simulink model "B5_simulation_paparazzi"  (R2021b)
settings: Solver=VariableStepAuto  StartTime=0.0  StopTime=5.5  FixedStep=0.002  RelTol=1e-3
values from neighbouring files (symbols this model uses):
  coef_sim_1 = tf_des_d.Denominator{1}(2)    [A11_setup_script_pprz.m]    (also in A1_setup_script.m; A6_slow_actuator.m)
  coef_sim_2 = tf_des_d.Numerator{1}(2)    [A11_setup_script_pprz.m]    (also in A1_setup_script.m; A6_slow_actuator.m)
  coeff = 1    [A11_setup_script_pprz.m]    (also in A12_sim_multi_run.m = coeff_list(i))
  doublet_mag = - 0.15    (= -0.15)    [A11_setup_script_pprz.m]    (also in A1_setup_script.m)
  doublet_time = 6    [A11_setup_script_pprz.m]    (also in A1_setup_script.m)
  f_8 = 1    [A11_setup_script_pprz.m]    (also in A1_setup_script.m)
  FILT_CUTOFF = 2*pi*5    (= 31.4159265359)    [A11_setup_script_pprz.m]    (also in A1_setup_script.m)
  FILTER = 1    [A11_setup_script_pprz.m]    (also in A1_setup_script.m)
  G1 = inv(I)*G1_r    [A10_simple_plant.m]    (also in A11_setup_script_pprz.m = G1/scale; A1_setup_script.m = [G1;G1_T])
  G2 = G2/scale    [A11_setup_script_pprz.m]    (also in A1_setup_script.m = (1/sampling_time)*inv(I)*(G2_r))
  h_plate = 0.3    [A11_setup_script_pprz.m]    (also in A1_setup_script.m = 0.16)
  I = eye(3,3)    [A10_simple_plant.m]    (also in A11_setup_script_pprz.m; A1_setup_script.m; A2_B_matrix_generation_symbolic.m = [Ixx 0 0; A3_B_matrix_generation_symbolic_cascaded.m = [Ixx 0 0)
  Iyy = 0.0008    [A11_setup_script_pprz.m]    (also in A1_setup_script.m = 0.0015)
  K = 7    [A11_setup_script_pprz.m]    (also in A1_setup_script.m = 10)
  K_act = 50    [A10_simple_plant.m]    (also in A11_setup_script_pprz.m = 20; A1_setup_script.m = 20)
  K_d = 15    [A11_setup_script_pprz.m]    (also in A1_setup_script.m = 25)
  K_dd = K_act    (= 20)    [A11_setup_script_pprz.m]    (also in A1_setup_script.m)
  K_ec = 50    [A11_setup_script_pprz.m]    (also in A1_setup_script.m = 251)
  K_ec_d = 13    [A11_setup_script_pprz.m]    (also in A1_setup_script.m = 25)
  K_ec_d_u = 1.5    [A11_setup_script_pprz.m]    (also in A1_setup_script.m = 5)
  K_ec_d_v = 1.5    [A11_setup_script_pprz.m]    (also in A1_setup_script.m = 5)
  K_ec_dd = 9    [A11_setup_script_pprz.m]    (also in A1_setup_script.m = 45)
  K_ec_i = 0    [A11_setup_script_pprz.m]    (also in A1_setup_script.m = 380)
  K_ec_u = 1.5    [A11_setup_script_pprz.m]    (also in A1_setup_script.m = 5)
  K_ec_v = 1.5    [A11_setup_script_pprz.m]    (also in A1_setup_script.m = 5)
  K_t = 0.0005    [A10_simple_plant.m]    (also in A11_setup_script_pprz.m = 6.557e-08; A1_setup_script.m = 6.557e-08)
  K_u = 1.0    (= 1)    [A11_setup_script_pprz.m]    (also in A1_setup_script.m = 1.5)
  K_u_d = 2.5    [A11_setup_script_pprz.m]    (also in A1_setup_script.m = 7)
  K_v = 1.0    (= 1)    [A11_setup_script_pprz.m]    (also in A1_setup_script.m = 1.5)
  K_v_d = 2.5    [A11_setup_script_pprz.m]    (also in A1_setup_script.m = 7)
  K_w = 1.0    (= 1)    [A11_setup_script_pprz.m]    (also in A1_setup_script.m = 4.5)
  K_w_d = 2.5    [A11_setup_script_pprz.m]    (also in A1_setup_script.m = 7)
  l_plate = 0.1    [A11_setup_script_pprz.m]    (also in A1_setup_script.m = 0.11)
  m = 0.4    [A10_simple_plant.m]    (also in A11_setup_script_pprz.m; A1_setup_script.m)
  NOISE = 0    [A11_setup_script_pprz.m]    (also in A1_setup_script.m)
  NOISE_ACC = 0.00005    (= 5e-05)    [A11_setup_script_pprz.m]    (also in A1_setup_script.m)
  NOISE_GYRO = 0.00005    (= 5e-05)    [A11_setup_script_pprz.m]    (also in A1_setup_script.m)
  NOISE_RPM = 200    [A11_setup_script_pprz.m]    (also in A1_setup_script.m)
  omega_des = 20.00    (= 20)    [A11_setup_script_pprz.m]    (also in A1_setup_script.m; A6_slow_actuator.m = 49)
  sampling_time = 1/frequency    (= 0.002)    [A11_setup_script_pprz.m]    (also in A12_sim_multi_run.m; A1_setup_script.m; A6_slow_actuator.m)
  scale_8 = 1.6    [A11_setup_script_pprz.m]    (also in A1_setup_script.m)
  start_8 = 2    [A11_setup_script_pprz.m]    (also in A1_setup_script.m)
  start_time = 2    [A11_setup_script_pprz.m]    (also in A1_setup_script.m = 1)
  t_8 = 10    [A11_setup_script_pprz.m]    (also in A1_setup_script.m)
  w_plate = 0.3    [A11_setup_script_pprz.m]    (also in A1_setup_script.m = 0.36)
undefined symbols (not defined in the file or in its folder): DiscIntNeverNeededParam
libraries: simulink x11, cstblocks x9, dspinverses x8, dspmathops x4, dspstat3 x4, aerolibutil x3, sharedutil x2, aerolibanim x1
(part 4 of 5)

== system B5_simulation_paparazzi/Model Block Complementary Filters/Plant and State Estimation/Complementary Filter1/Butterworth Lowpass 2nd Order1 ==
  In : Inport
  Constant : Constant  Value=FILTER  SampleTime=sampling_time
  Merge : Merge
  Switch Case : SwitchCase
  Switch Case Action Subsystem : Subsystem  TreatAsAtomicUnit=on
  Switch Case Action Subsystem1 : Subsystem  TreatAsAtomicUnit=on
  Out : Outport
  wires:
  Merge/1 -> Out/1
  Switch Case Action Subsystem/1(Out1) -> Merge/1
  Constant/1 -> Switch Case/1
  Switch Case Action Subsystem1/1(Out1) -> Merge/2
  Switch Case/2 -> Switch Case Action Subsystem1/Action
  In/1 -> Switch Case Action Subsystem/1(In1), Switch Case Action Subsystem1/1(In1)
  Switch Case/1 -> Switch Case Action Subsystem/Action

== system B5_simulation_paparazzi/Model Block Complementary Filters/Plant and State Estimation/Complementary Filter1/Butterworth Lowpass 2nd Order2 ==
  In : Inport
  Constant : Constant  Value=FILTER  SampleTime=sampling_time
  Merge : Merge
  Switch Case : SwitchCase
  Switch Case Action Subsystem : Subsystem  TreatAsAtomicUnit=on
  Switch Case Action Subsystem1 : Subsystem  TreatAsAtomicUnit=on
  Out : Outport
  wires:
  Merge/1 -> Out/1
  Switch Case Action Subsystem/1(Out1) -> Merge/1
  Constant/1 -> Switch Case/1
  Switch Case Action Subsystem1/1(Out1) -> Merge/2
  Switch Case/2 -> Switch Case Action Subsystem1/Action
  In/1 -> Switch Case Action Subsystem/1(In1), Switch Case Action Subsystem1/1(In1)
  Switch Case/1 -> Switch Case Action Subsystem/Action

== system B5_simulation_paparazzi/Model Block Complementary Filters/Plant and State Estimation/Noise Acc/Switch Case Action Subsystem ==
  Action Port : ActionPort  ActionPortLabel=case [ 1 ]:
  Acc Noise : simulink/Sources/Band-Limited White Noise  Cov=[NOISE_ACC]  Ts=sampling_time  seed=[23341]
  Out1 : Outport
  wires:
  Acc Noise/1 -> Out1/1

== system B5_simulation_paparazzi/Model Block Complementary Filters/Plant and State Estimation/Noise Acc/Switch Case Action Subsystem1 ==
  Action Port : ActionPort  ActionPortLabel=default:
  Constant : Constant  Value=0  SampleTime=sampling_time
  Out1 : Outport
  wires:
  Constant/1 -> Out1/1

== system B5_simulation_paparazzi/Model Block Complementary Filters/Plant and State Estimation/Noise Gyro/Switch Case Action Subsystem ==
  Action Port : ActionPort  ActionPortLabel=case [ 1 ]:
  Gyro Noise : simulink/Sources/Band-Limited White Noise  Cov=[NOISE_GYRO]  Ts=sampling_time  seed=[23341]
  Out1 : Outport
  wires:
  Gyro Noise/1 -> Out1/1

== system B5_simulation_paparazzi/Model Block Complementary Filters/Plant and State Estimation/Noise Gyro/Switch Case Action Subsystem1 ==
  Action Port : ActionPort  ActionPortLabel=default:
  Constant : Constant  Value=0  SampleTime=sampling_time
  Out1 : Outport
  wires:
  Constant/1 -> Out1/1

== system B5_simulation_paparazzi/Model Block Complementary Filters/Plant and State Estimation/Plant Dynamics Continuous/Disturbance Block ==
  Step : Step  Time=2  After=60  SampleTime=0
  Sum : Sum  Inputs=|++
  Total Disturbance : Outport
  wires:
  Step/1 -> Sum/1
  Sum/1 -> Total Disturbance/1

== system B5_simulation_paparazzi/Model Block Complementary Filters/Plant and State Estimation/Plant Dynamics Continuous/Omega_I_Omega1 ==
  pqr_body : Inport
  Inertia : Inport  Port=2
  3x3 Cross Product : sharedutil/3x3 Cross Product  aMode=aMode
      settings: SourceProductBaseCode=AE,PW,DR,MT,UV,VE
  Matrix Multiply1 : Product  Multiplication=Matrix(*)
  Final product : Outport
  wires:
  Inertia/1 -> Matrix Multiply1/1
  Matrix Multiply1/1 -> 3x3 Cross Product/2
  3x3 Cross Product/1 -> Final product/1
  pqr_body/1 -> 3x3 Cross Product/1, Matrix Multiply1/2

== system B5_simulation_paparazzi/Model Block Complementary Filters/Simple INDI/INTERNAL REFERENCE MODEL ATTITUDE/body rates to euler rates ==
  p : Inport
  q : Inport  Port=2
  r : Inport  Port=3
  Demux : Demux  Outputs=3
  Matrix Multiply : Product  Multiplication=Matrix(*)
  Mux : Mux  Inputs=3
  phi_dot : Outport
  theta_dot : Outport  Port=2
  psi_dot : Outport  Port=3
  wires:
  p/1 -> Mux/1
  q/1 -> Mux/2
  r/1 -> Mux/3
  [T_discr] -> Matrix Multiply/1
  Mux/1 -> Matrix Multiply/2
  Matrix Multiply/1 -> Demux/1
  Demux/3 -> psi_dot/1
  Demux/2 -> theta_dot/1
  Demux/1 -> phi_dot/1

== system B5_simulation_paparazzi/Model Block Complementary Filters/Simple INDI/INTERNAL REFERENCE MODEL ATTITUDE/euler rates to body rates ==
  phi_dot : Inport
  theta_dot : Inport  Port=2
  psi_dot : Inport  Port=3
  Demux : Demux  Outputs=3
  Matrix Multiply : Product  Multiplication=Matrix(*)
  Mux : Mux  Inputs=3
  p : Outport
  q : Outport  Port=2
  r : Outport  Port=3
  wires:
  phi_dot/1 -> Mux/1
  theta_dot/1 -> Mux/2
  psi_dot/1 -> Mux/3
  [R_discr] -> Matrix Multiply/1
  Mux/1 -> Matrix Multiply/2
  Matrix Multiply/1 -> Demux/1
  Demux/3 -> r/1
  Demux/2 -> q/1
  Demux/1 -> p/1

== system B5_simulation_paparazzi/Model Block Normal Filters/Continuous Actuator Dynamics/Butterworth Lowpass 2nd Order1/Switch Case Action Subsystem ==
  In1 : Inport
  Action Port : ActionPort  ActionPortLabel=case [ 1 ]:
  Constant5 : Constant  Value=FILT_CUTOFF  SampleTime=sampling_time
  Lowpass2 : cstblocks/Linear Parameter Varying/Discrete Varying Lowpass  N=2  w0=0  Ts=sampling_time
      settings: SourceProductBaseCode=CT
  Out1 : Outport
  wires:
  Constant5/1 -> Lowpass2/2
  In1/1 -> Lowpass2/1
  Lowpass2/1 -> Out1/1

== system B5_simulation_paparazzi/Model Block Normal Filters/Continuous Actuator Dynamics/Butterworth Lowpass 2nd Order1/Switch Case Action Subsystem1 ==
  In1 : Inport
  Action Port : ActionPort  ActionPortLabel=default:
  Out1 : Outport
  wires:
  In1/1 -> Out1/1

== system B5_simulation_paparazzi/Model Block Normal Filters/Continuous Actuator Dynamics/Noise RPM/Switch Case Action Subsystem ==
  Action Port : ActionPort  ActionPortLabel=case [ 1 ]:
  RPM Noise : simulink/Sources/Band-Limited White Noise  Cov=[NOISE_RPM]  Ts=sampling_time  seed=[23341]
  Out1 : Outport
  wires:
  RPM Noise/1 -> Out1/1

== system B5_simulation_paparazzi/Model Block Normal Filters/Continuous Actuator Dynamics/Noise RPM/Switch Case Action Subsystem1 ==
  Action Port : ActionPort  ActionPortLabel=default:
  Constant : Constant  Value=0  SampleTime=sampling_time
  Out1 : Outport
  wires:
  Constant/1 -> Out1/1

== system B5_simulation_paparazzi/Model Block Normal Filters/Extended INDI/INTERNAL REFERENCE MODEL ATTITUDE/body rates to euler rates ==
  p : Inport
  q : Inport  Port=2
  r : Inport  Port=3
  Demux : Demux  Outputs=3
  Matrix Multiply : Product  Multiplication=Matrix(*)
  Mux : Mux  Inputs=3
  phi_dot : Outport
  theta_dot : Outport  Port=2
  psi_dot : Outport  Port=3
  wires:
  p/1 -> Mux/1
  q/1 -> Mux/2
  r/1 -> Mux/3
  [T_discr] -> Matrix Multiply/1
  Mux/1 -> Matrix Multiply/2
  Matrix Multiply/1 -> Demux/1
  Demux/3 -> psi_dot/1
  Demux/2 -> theta_dot/1
  Demux/1 -> phi_dot/1

== system B5_simulation_paparazzi/Model Block Normal Filters/Extended INDI/INTERNAL REFERENCE MODEL ATTITUDE/euler rates to body rates ==
  phi_dot : Inport
  theta_dot : Inport  Port=2
  psi_dot : Inport  Port=3
  Demux : Demux  Outputs=3
  Matrix Multiply : Product  Multiplication=Matrix(*)
  Mux : Mux  Inputs=3
  p : Outport
  q : Outport  Port=2
  r : Outport  Port=3
  wires:
  phi_dot/1 -> Mux/1
  theta_dot/1 -> Mux/2
  psi_dot/1 -> Mux/3
  [R_discr] -> Matrix Multiply/1
  Mux/1 -> Matrix Multiply/2
  Matrix Multiply/1 -> Demux/1
  Demux/3 -> r/1
  Demux/2 -> q/1
  Demux/1 -> p/1

== system B5_simulation_paparazzi/Model Block Normal Filters/Extended INDI/Subsystem/body rates to euler rates ==
  p : Inport
  q : Inport  Port=2
  r : Inport  Port=3
  Demux : Demux  Outputs=3
  Matrix Multiply : Product  Multiplication=Matrix(*)
  Mux : Mux  Inputs=3
  phi_dot : Outport
  theta_dot : Outport  Port=2
  psi_dot : Outport  Port=3
  wires:
  p/1 -> Mux/1
  q/1 -> Mux/2
  r/1 -> Mux/3
  [T_discr] -> Matrix Multiply/1
  Mux/1 -> Matrix Multiply/2
  Matrix Multiply/1 -> Demux/1
  Demux/3 -> psi_dot/1
  Demux/2 -> theta_dot/1
  Demux/1 -> phi_dot/1

== system B5_simulation_paparazzi/Model Block Normal Filters/Plant and State Estimation/Butterworth Lowpass 2nd Order1/Switch Case Action Subsystem ==
  In1 : Inport
  Action Port : ActionPort  ActionPortLabel=case [ 1 ]:
  Constant5 : Constant  Value=FILT_CUTOFF  SampleTime=sampling_time
  Lowpass2 : cstblocks/Linear Parameter Varying/Discrete Varying Lowpass  N=2  w0=0  Ts=sampling_time
      settings: SourceProductBaseCode=CT
  Out1 : Outport
  wires:
  Constant5/1 -> Lowpass2/2
  In1/1 -> Lowpass2/1
  Lowpass2/1 -> Out1/1

== system B5_simulation_paparazzi/Model Block Normal Filters/Plant and State Estimation/Butterworth Lowpass 2nd Order1/Switch Case Action Subsystem1 ==
  In1 : Inport
  Action Port : ActionPort  ActionPortLabel=default:
  Out1 : Outport
  wires:
  In1/1 -> Out1/1

== system B5_simulation_paparazzi/Model Block Normal Filters/Plant and State Estimation/Butterworth Lowpass 2nd Order2/Switch Case Action Subsystem ==
  In1 : Inport
  Action Port : ActionPort  ActionPortLabel=case [ 1 ]:
  Constant5 : Constant  Value=FILT_CUTOFF  SampleTime=sampling_time
  Lowpass2 : cstblocks/Linear Parameter Varying/Discrete Varying Lowpass  N=2  w0=0  Ts=sampling_time
      settings: SourceProductBaseCode=CT
  Out1 : Outport
  wires:
  Constant5/1 -> Lowpass2/2
  In1/1 -> Lowpass2/1
  Lowpass2/1 -> Out1/1

== system B5_simulation_paparazzi/Model Block Normal Filters/Plant and State Estimation/Butterworth Lowpass 2nd Order2/Switch Case Action Subsystem1 ==
  In1 : Inport
  Action Port : ActionPort  ActionPortLabel=default:
  Out1 : Outport
  wires:
  In1/1 -> Out1/1

== system B5_simulation_paparazzi/Model Block Normal Filters/Plant and State Estimation/Butterworth Lowpass 2nd Order3/Switch Case Action Subsystem ==
  In1 : Inport
  Action Port : ActionPort
  Constant5 : Constant  Value=FILT_CUTOFF  SampleTime=sampling_time
  Lowpass2 : cstblocks/Linear Parameter Varying/Discrete Varying Lowpass  N=2  w0=0  Ts=sampling_time
      settings: SourceProductBaseCode=CT
  Out1 : Outport
  wires:
  Constant5/1 -> Lowpass2/2
  In1/1 -> Lowpass2/1
  Lowpass2/1 -> Out1/1

== system B5_simulation_paparazzi/Model Block Normal Filters/Plant and State Estimation/Butterworth Lowpass 2nd Order3/Switch Case Action Subsystem1 ==
  In1 : Inport
  Action Port : ActionPort
  Out1 : Outport
  wires:
  In1/1 -> Out1/1

== system B5_simulation_paparazzi/Model Block Normal Filters/Plant and State Estimation/Butterworth Lowpass 2nd Order4/Switch Case Action Subsystem ==
  In1 : Inport
  Action Port : ActionPort
  Constant5 : Constant  Value=FILT_CUTOFF  SampleTime=sampling_time
  Lowpass2 : cstblocks/Linear Parameter Varying/Discrete Varying Lowpass  N=2  w0=0  Ts=sampling_time
      settings: SourceProductBaseCode=CT
  Out1 : Outport
  wires:
  Constant5/1 -> Lowpass2/2
  In1/1 -> Lowpass2/1
  Lowpass2/1 -> Out1/1

== system B5_simulation_paparazzi/Model Block Normal Filters/Plant and State Estimation/Butterworth Lowpass 2nd Order4/Switch Case Action Subsystem1 ==
  In1 : Inport
  Action Port : ActionPort
  Out1 : Outport
  wires:
  In1/1 -> Out1/1

== system B5_simulation_paparazzi/Model Block Normal Filters/Plant and State Estimation/Noise Acc/Switch Case Action Subsystem ==
  Action Port : ActionPort  ActionPortLabel=case [ 1 ]:
  Acc Noise : simulink/Sources/Band-Limited White Noise  Cov=[NOISE_ACC]  Ts=sampling_time  seed=[23341]
  Out1 : Outport
  wires:
  Acc Noise/1 -> Out1/1

== system B5_simulation_paparazzi/Model Block Normal Filters/Plant and State Estimation/Noise Acc/Switch Case Action Subsystem1 ==
  Action Port : ActionPort  ActionPortLabel=default:
  Constant : Constant  Value=0  SampleTime=sampling_time
  Out1 : Outport
  wires:
  Constant/1 -> Out1/1

== system B5_simulation_paparazzi/Model Block Normal Filters/Plant and State Estimation/Noise Gyro/Switch Case Action Subsystem ==
  Action Port : ActionPort  ActionPortLabel=case [ 1 ]:
  Gyro Noise : simulink/Sources/Band-Limited White Noise  Cov=[NOISE_GYRO]  Ts=sampling_time  seed=[23341]
  Out1 : Outport
  wires:
  Gyro Noise/1 -> Out1/1

== system B5_simulation_paparazzi/Model Block Normal Filters/Plant and State Estimation/Noise Gyro/Switch Case Action Subsystem1 ==
  Action Port : ActionPort  ActionPortLabel=default:
  Constant : Constant  Value=0  SampleTime=sampling_time
  Out1 : Outport
  wires:
  Constant/1 -> Out1/1

== system B5_simulation_paparazzi/Model Block Normal Filters/Plant and State Estimation/Plant Dynamics Continuous/Disturbance Block ==
  Step : Step  Time=2  After=60  SampleTime=0
  Sum : Sum  Inputs=|++
  Total Disturbance : Outport
  wires:
  Step/1 -> Sum/1
  Sum/1 -> Total Disturbance/1

== system B5_simulation_paparazzi/Model Block Normal Filters/Plant and State Estimation/Plant Dynamics Continuous/Omega_I_Omega1 ==
  pqr_body : Inport
  Inertia : Inport  Port=2
  3x3 Cross Product : sharedutil/3x3 Cross Product  aMode=aMode
      settings: SourceProductBaseCode=AE,PW,DR,MT,UV,VE
  Matrix Multiply1 : Product  Multiplication=Matrix(*)
  Final product : Outport
  wires:
  Inertia/1 -> Matrix Multiply1/1
  Matrix Multiply1/1 -> 3x3 Cross Product/2
  3x3 Cross Product/1 -> Final product/1
  pqr_body/1 -> 3x3 Cross Product/1, Matrix Multiply1/2

== system B5_simulation_paparazzi/Model Block Normal Filters/Simple INDI/INTERNAL REFERENCE MODEL ATTITUDE/body rates to euler rates ==
  p : Inport
  q : Inport  Port=2
  r : Inport  Port=3
  Demux : Demux  Outputs=3
  Matrix Multiply : Product  Multiplication=Matrix(*)
  Mux : Mux  Inputs=3
  phi_dot : Outport
  theta_dot : Outport  Port=2
  psi_dot : Outport  Port=3
  wires:
  p/1 -> Mux/1
  q/1 -> Mux/2
  r/1 -> Mux/3
  [T_discr] -> Matrix Multiply/1
  Mux/1 -> Matrix Multiply/2
  Matrix Multiply/1 -> Demux/1
  Demux/3 -> psi_dot/1
  Demux/2 -> theta_dot/1
  Demux/1 -> phi_dot/1

== system B5_simulation_paparazzi/Model Block Normal Filters/Simple INDI/INTERNAL REFERENCE MODEL ATTITUDE/euler rates to body rates ==
  phi_dot : Inport
  theta_dot : Inport  Port=2
  psi_dot : Inport  Port=3
  Demux : Demux  Outputs=3
  Matrix Multiply : Product  Multiplication=Matrix(*)
  Mux : Mux  Inputs=3
  p : Outport
  q : Outport  Port=2
  r : Outport  Port=3
  wires:
  phi_dot/1 -> Mux/1
  theta_dot/1 -> Mux/2
  psi_dot/1 -> Mux/3
  [R_discr] -> Matrix Multiply/1
  Mux/1 -> Matrix Multiply/2
  Matrix Multiply/1 -> Demux/1
  Demux/3 -> r/1
  Demux/2 -> q/1
  Demux/1 -> p/1

== system B5_simulation_paparazzi/Model Block Complementary Filters/Plant and State Estimation/Complementary Filter/Butterworth Lowpass 2nd Order1/Switch Case Action Subsystem ==
  In1 : Inport
  Action Port : ActionPort  ActionPortLabel=case [ 1 ]:
  Constant5 : Constant  Value=FILT_CUTOFF  SampleTime=sampling_time
  Lowpass2 : cstblocks/Linear Parameter Varying/Discrete Varying Lowpass  N=2  w0=0  Ts=sampling_time
      settings: SourceProductBaseCode=CT
  Out1 : Outport
  wires:
  Constant5/1 -> Lowpass2/2
  In1/1 -> Lowpass2/1
  Lowpass2/1 -> Out1/1

== system B5_simulation_paparazzi/Model Block Complementary Filters/Plant and State Estimation/Complementary Filter/Butterworth Lowpass 2nd Order1/Switch Case Action Subsystem1 ==
  In1 : Inport
  Action Port : ActionPort  ActionPortLabel=default:
  Out1 : Outport
  wires:
  In1/1 -> Out1/1

== system B5_simulation_paparazzi/Model Block Complementary Filters/Plant and State Estimation/Complementary Filter/Butterworth Lowpass 2nd Order2/Switch Case Action Subsystem ==
  In1 : Inport
  Action Port : ActionPort  ActionPortLabel=case [ 1 ]:
  Constant5 : Constant  Value=FILT_CUTOFF  SampleTime=sampling_time
  Lowpass2 : cstblocks/Linear Parameter Varying/Discrete Varying Lowpass  N=2  w0=0  Ts=sampling_time
      settings: SourceProductBaseCode=CT
  Out1 : Outport
  wires:
  Constant5/1 -> Lowpass2/2
  In1/1 -> Lowpass2/1
  Lowpass2/1 -> Out1/1

== system B5_simulation_paparazzi/Model Block Complementary Filters/Plant and State Estimation/Complementary Filter/Butterworth Lowpass 2nd Order2/Switch Case Action Subsystem1 ==
  In1 : Inport
  Action Port : ActionPort  ActionPortLabel=default:
  Out1 : Outport
  wires:
  In1/1 -> Out1/1

== system B5_simulation_paparazzi/Model Block Complementary Filters/Plant and State Estimation/Complementary Filter1/Butterworth Lowpass 2nd Order1/Switch Case Action Subsystem ==
  In1 : Inport
  Action Port : ActionPort  ActionPortLabel=case [ 1 ]:
  Constant5 : Constant  Value=FILT_CUTOFF  SampleTime=sampling_time
  Lowpass2 : cstblocks/Linear Parameter Varying/Discrete Varying Lowpass  N=2  w0=0  Ts=sampling_time
      settings: SourceProductBaseCode=CT
  Out1 : Outport
  wires:
  Constant5/1 -> Lowpass2/2
  In1/1 -> Lowpass2/1
  Lowpass2/1 -> Out1/1

== system B5_simulation_paparazzi/Model Block Complementary Filters/Plant and State Estimation/Complementary Filter1/Butterworth Lowpass 2nd Order1/Switch Case Action Subsystem1 ==
  In1 : Inport
  Action Port : ActionPort  ActionPortLabel=default:
  Out1 : Outport
  wires:
  In1/1 -> Out1/1

== system B5_simulation_paparazzi/Model Block Complementary Filters/Plant and State Estimation/Complementary Filter1/Butterworth Lowpass 2nd Order2/Switch Case Action Subsystem ==
  In1 : Inport
  Action Port : ActionPort  ActionPortLabel=case [ 1 ]:
  Constant5 : Constant  Value=FILT_CUTOFF  SampleTime=sampling_time
  Lowpass2 : cstblocks/Linear Parameter Varying/Discrete Varying Lowpass  N=2  w0=0  Ts=sampling_time
      settings: SourceProductBaseCode=CT
  Out1 : Outport
  wires:
  Constant5/1 -> Lowpass2/2
  In1/1 -> Lowpass2/1
  Lowpass2/1 -> Out1/1

== system B5_simulation_paparazzi/Model Block Complementary Filters/Plant and State Estimation/Complementary Filter1/Butterworth Lowpass 2nd Order2/Switch Case Action Subsystem1 ==
  In1 : Inport
  Action Port : ActionPort  ActionPortLabel=default:
  Out1 : Outport
  wires:
  In1/1 -> Out1/1

== matlab function B5_simulation_paparazzi/Model Block Complementary Filters/Simple INDI/8-shape trajectory/MATLAB Function ==
  data: x output; t input; y output; f input; scale input; psi output; sampling_time input; total_time input; start_time input
function [x,y,psi] = inf_trajectory(t,f,scale,sampling_time,total_time,start_time)

t_norm = t/total_time;

x = 2*scale*sin(2*pi*f*t_norm);
y = scale*sin(2*pi*f*t_norm*2);

x_n = 2*scale*sin(2*pi*f*(t_norm+sampling_time));
y_n = scale*sin(2*pi*f*(t_norm+sampling_time)*2);

dx = x_n - x;
dy = y_n - y;

psi = atan2(dy,dx);

== matlab function B5_simulation_paparazzi/Model Block Complementary Filters/Simple INDI/ERROR CONTROLLER ATTITUDE/MATLAB Function1 ==
  data: pis_e input; psie_w output
function psie_w = wrapper(pis_e)

if pis_e > pi
    psie_w = pis_e - 2*pi;
elseif pis_e <= -pi
    psie_w = pis_e + 2*pi;
else
    psie_w = pis_e;
end

== matlab function B5_simulation_paparazzi/Model Block Complementary Filters/Simple INDI/G1+G2 ==
  data: G1 input; B_inner output; G2 input
function B_inner = B_inner(G1,G2)

% add additional row to G2 for equal size
G2_T = [0 0 0 0];
G2 = vertcat(G2,G2_T);

% B_inner = K_act*(G1 + G2);
B_inner = G1;

== matlab function B5_simulation_paparazzi/Model Block Complementary Filters/Simple INDI/G2_comp ==
  data: G2 input; domega input; G2_comp output
function G2_comp = G2_comp(G2,domega)

G2_comp = G2(3,:) * domega;

== matlab function B5_simulation_paparazzi/Model Block Complementary Filters/Simple INDI/INTERNAL REFERENCE MODEL ATTITUDE/MATLAB Function1 ==
  data: pis_e input; psie_w output
function psie_w = wrapper(pis_e)

if pis_e > pi
    psie_w = pis_e - 2*pi;
elseif pis_e <= -pi
    psie_w = pis_e + 2*pi;
else
    psie_w = pis_e;
end

== matlab function B5_simulation_paparazzi/Model Block Complementary Filters/Simple INDI/MATLAB Function1 ==
  data: T input; B_outer output; Phi input; Theta input; Psi input; m input
function B_outer = control_allocation_simple_outer(T,Phi,Theta,Psi,m)

B_outer = zeros(3,3);

% matrix obtained in ZXY rotation
% output order u = [phi theta thrust]
B_outer(1,1) = (T*cos(Phi)*cos(Psi)*cos(Theta))/m;
B_outer(2,1) = (T*cos(Phi)*cos(Theta)*sin(Psi))/m;
B_outer(3,1) = -(T*cos(Phi)*sin(Theta))/m;

B_outer(1,2) = (T*(cos(Phi)*sin(Psi) - cos(Psi)*sin(Phi)*sin(Theta)))/m;
B_outer(2,2) = -(T*(cos(Phi)*cos(Psi) + sin(Phi)*sin(Psi)*sin(Theta)))/m;
B_outer(3,2) = -(T*cos(Theta)*sin(Phi))/m;

B_outer(1,3) = (sin(Phi)*sin(Psi) + cos(Phi)*cos(Psi)*sin(Theta))/m;
B_outer(2,3) = -(cos(Psi)*sin(Phi) - cos(Phi)*sin(Psi)*sin(Theta))/m;
B_outer(3,3) = (cos(Phi)*cos(Theta))/m;

end

== matlab function B5_simulation_paparazzi/Model Block Normal Filters/Extended INDI/8-shape trajectory/MATLAB Function ==
  data: x output; t input; y output; f input; scale input; psi output; sampling_time input; total_time input; start_time input
function [x,y,psi] = inf_trajectory(t,f,scale,sampling_time,total_time,start_time)

t_norm = t/total_time;

x = 2*scale*sin(2*pi*f*t_norm);
y = scale*sin(2*pi*f*t_norm*2);

x_n = 2*scale*sin(2*pi*f*(t_norm+sampling_time));
y_n = scale*sin(2*pi*f*(t_norm+sampling_time)*2);

dx = x_n - x;
dy = y_n - y;

psi = atan2(dy,dx);

== matlab function B5_simulation_paparazzi/Model Block Normal Filters/Extended INDI/ERROR CONTROLLER ATTITUDE/MATLAB Function1 ==
  data: pis_e input; psie_w output
function psie_w = wrapper(pis_e)

if pis_e > pi
    psie_w = pis_e - 2*pi;
elseif pis_e <= -pi
    psie_w = pis_e + 2*pi;
else
    psie_w = pis_e;
end

== matlab function B5_simulation_paparazzi/Model Block Normal Filters/Extended INDI/G1+G2 ==
  data: G1 input; B_inner output; G2 input; K_act input
function B_inner = B_inner(G1,G2,K_act)

% add additional row to G2 for equal size
G2_T = [0 0 0 0];
G2 = vertcat(G2,G2_T);

% B_inner = K_act*(G1 + G2);
B_inner = K_act*(G1);

== matlab function B5_simulation_paparazzi/Model Block Normal Filters/Extended INDI/G2_comp ==
  data: G2 input; K_act input; domega input; G2_comp output
function G2_comp = G2_comp(G2,K_act,domega)

G2_comp = K_act * G2(3,:) * domega;

== matlab function B5_simulation_paparazzi/Model Block Normal Filters/Extended INDI/INTERNAL REFERENCE MODEL ATTITUDE/MATLAB Function1 ==
  data: pis_e input; psie_w output
function psie_w = wrapper(pis_e)

if pis_e > pi
    psie_w = pis_e - 2*pi;
elseif pis_e <= -pi
    psie_w = pis_e + 2*pi;
else
    psie_w = pis_e;
end

== matlab function B5_simulation_paparazzi/Model Block Normal Filters/Extended INDI/MATLAB Function1 ==
  data: T input; B_outer output; Phi input; Theta input; Psi input; m input
function B_outer = control_allocation_simple_outer(T,Phi,Theta,Psi,m)

B_outer = zeros(3,3);

% matrix obtained in ZXY rotation
% output order u = [phi theta thrust]
B_outer(1,1) = (T*cos(Phi)*cos(Psi)*cos(Theta))/m;
B_outer(2,1) = (T*cos(Phi)*cos(Theta)*sin(Psi))/m;
B_outer(3,1) = -(T*cos(Phi)*sin(Theta))/m;

B_outer(1,2) = (T*(cos(Phi)*sin(Psi) - cos(Psi)*sin(Phi)*sin(Theta)))/m;
B_outer(2,2) = -(T*(cos(Phi)*cos(Psi) + sin(Phi)*sin(Psi)*sin(Theta)))/m;
B_outer(3,2) = -(T*cos(Theta)*sin(Phi))/m;

B_outer(1,3) = (sin(Phi)*sin(Psi) + cos(Phi)*cos(Psi)*sin(Theta))/m;
B_outer(2,3) = -(cos(Psi)*sin(Phi) - cos(Phi)*sin(Psi)*sin(Theta))/m;
B_outer(3,3) = (cos(Phi)*cos(Theta))/m;

end

== matlab function B5_simulation_paparazzi/Model Block Normal Filters/Extended INDI/Subsystem/MATLAB Function ==
  data: theta input; qdd_comp output; dtheta input; Vx input; Vy input; Vz input; Ax input; Ay input; Az input; u input; w_plate input; h_plate input; l_plate input; Iyy input
function qdd_comp = fcn(theta,dtheta,Vx,Vy,Vz,Ax,Ay,Az,u,w_plate,h_plate,l_plate,Iyy)

S_plate = w_plate * h_plate;
rho = 1.225;
Cd1 = 0.0033;
Cd2 = 0.7;
Cl1 = -0.0228;
Cl2 = 2.01;

% Cd = + 0.7 (correct)
qdd_comp = - (dtheta*l_plate*sign(u)*((S_plate*rho*cos((pi*((180*theta)/pi + (180*atan2(Vz, (Vx^2 + Vy^2)^(1/2)))/pi))/180)*(Cl2 + Cl1*((180*theta)/pi + (180*atan2(Vz, (Vx^2 + Vy^2)^(1/2)))/pi + 90))*(Vx^2 + Vy^2 + Vz^2))/2 + (S_plate*rho*sin((pi*((180*theta)/pi + (180*atan2(Vz, (Vx^2 + Vy^2)^(1/2)))/pi))/180)*(Cd2 + Cd1*((180*theta)/pi + (180*atan2(Vz, (Vx^2 + Vy^2)^(1/2)))/pi + 90))*(Vx^2 + Vy^2 + Vz^2))/2 - (90*Cd1*S_plate*rho*cos((pi*((180*theta)/pi + (180*atan2(Vz, (Vx^2 + Vy^2)^(1/2)))/pi))/180)*(Vx^2 + Vy^2 + Vz^2))/pi + (90*Cl1*S_plate*rho*sin((pi*((180*theta)/pi + (180*atan2(Vz, (Vx^2 + Vy^2)^(1/2)))/pi))/180)*(Vx^2 + Vy^2 + Vz^2))/pi))/Iyy + (Ax*l_plate*sign(u)*(- S_plate*Vx*rho*sin((pi*((180*theta)/pi + (180*atan2(Vz, (Vx^2 + Vy^2)^(1/2)))/pi))/180)*(Cl2 + Cl1*((180*theta)/pi + (180*atan2(Vz, (Vx^2 + Vy^2)^(1/2)))/pi + 90)) + S_plate*Vx*rho*cos((pi*((180*theta)/pi + (180*atan2(Vz, (Vx^2 + Vy^2)^(1/2)))/pi))/180)*(Cd2 + Cd1*((180*theta)/pi + (180*atan2(Vz, (Vx^2 + Vy^2)^(1/2)))/pi + 90)) + (S_plate*Vx*Vz*rho*cos((pi*((180*theta)/pi + (180*atan2(Vz, (Vx^2 + Vy^2)^(1/2)))/pi))/180)*(Cl2 + Cl1*((180*theta)/pi + (180*atan2(Vz, (Vx^2 + Vy^2)^(1/2)))/pi + 90)))/(2*(Vx^2 + Vy^2)^(1/2)) + (S_plate*Vx*Vz*rho*sin((pi*((180*theta)/pi + (180*atan2(Vz, (Vx^2 + Vy^2)^(1/2)))/pi))/180)*(Cd2 + Cd1*((180*theta)/pi + (180*atan2(Vz, (Vx^2 + Vy^2)^(1/2)))/pi + 90)))/(2*(Vx^2 + Vy^2)^(1/2)) - (90*Cd1*S_plate*Vx*Vz*rho*cos((pi*((180*theta)/pi + (180*atan2(Vz, (Vx^2 + Vy^2)^(1/2)))/pi))/180))/(pi*(Vx^2 + Vy^2)^(1/2)) + (90*Cl1*S_plate*Vx*Vz*rho*sin((pi*((180*theta)/pi + (180*atan2(Vz, (Vx^2 + Vy^2)^(1/2)))/pi))/180))/(pi*(Vx^2 + Vy^2)^(1/2))))/Iyy + (Ay*l_plate*sign(u)*(- S_plate*Vy*rho*sin((pi*((180*theta)/pi + (180*atan2(Vz, (Vx^2 + Vy^2)^(1/2)))/pi))/180)*(Cl2 + Cl1*((180*theta)/pi + (180*atan2(Vz, (Vx^2 + Vy^2)^(1/2)))/pi + 90)) + S_plate*Vy*rho*cos((pi*((180*theta)/pi + (180*atan2(Vz, (Vx^2 + Vy^2)^(1/2)))/pi))/180)*(Cd2 + Cd1*((180*theta)/pi + (180*atan2(Vz, (Vx^2 + Vy^2)^(1/2)))/pi + 90)) + (S_plate*Vy*Vz*rho*cos((pi*((180*theta)/pi + (180*atan2(Vz, (Vx^2 + Vy^2)^(1/2)))/pi))/180)*(Cl2 + Cl1*((180*theta)/pi + (180*atan2(Vz, (Vx^2 + Vy^2)^(1/2)))/pi + 90)))/(2*(Vx^2 + Vy^2)^(1/2)) + (S_plate*Vy*Vz*rho*sin((pi*((180*theta)/pi + (180*atan2(Vz, (Vx^2 + Vy^2)^(1/2)))/pi))/180)*(Cd2 + Cd1*((180*theta)/pi + (180*atan2(Vz, (Vx^2 + Vy^2)^(1/2)))/pi + 90)))/(2*(Vx^2 + Vy^2)^(1/2)) - (90*Cd1*S_plate*Vy*Vz*rho*cos((pi*((180*theta)/pi + (180*atan2(Vz, (Vx^2 + Vy^2)^(1/2)))/pi))/180))/(pi*(Vx^2 + Vy^2)^(1/2)) + (90*Cl1*S_plate*Vy*Vz*rho*sin((pi*((180*theta)/pi + (180*atan2(Vz, (Vx^2 + Vy^2)^(1/2)))/pi))/180))/(pi*(Vx^2 + Vy^2)^(1/2))))/Iyy - (Az*l_plate*sign(u)*(S_plate*Vz*rho*sin((pi*((180*theta)/pi + (180*atan2(Vz, (Vx^2 + Vy^2)^(1/2)))/pi))/180)*(Cl2 + Cl1*((180*theta)/pi + (180*atan2(Vz, (Vx^2 + Vy^2)^(1/2)))/pi + 90)) + (S_plate*rho*cos((pi*((180*theta)/pi + (180*atan2(Vz, (Vx^2 + Vy^2)^(1/2)))/pi))/180)*(Vx^2 + Vy^2)^(1/2)*(Cl2 + Cl1*((180*theta)/pi + (180*atan2(Vz, (Vx^2 + Vy^2)^(1/2)))/pi + 90)))/2 + (S_plate*rho*sin((pi*((180*theta)/pi + (180*atan2(Vz, (Vx^2 + Vy^2)^(1/2)))/pi))/180)*(Vx^2 + Vy^2)^(1/2)*(Cd2 + Cd1*((180*theta)/pi + (180*atan2(Vz, (Vx^2 + Vy^2)^(1/2)))/pi + 90)))/2 - S_plate*Vz*rho*cos((pi*((180*theta)/pi + (180*atan2(Vz, (Vx^2 + Vy^2)^(1/2)))/pi))/180)*(Cd2 + Cd1*((180*theta)/pi + (180*atan2(Vz, (Vx^2 + Vy^2)^(1/2)))/pi + 90)) - (90*Cd1*S_plate*rho*cos((pi*((180*theta)/pi + (180*atan2(Vz, (Vx^2 + Vy^2)^(1/2)))/pi))/180)*(Vx^2 + Vy^2)^(1/2))/pi + (90*Cl1*S_plate*rho*sin((pi*((180*theta)/pi + (180*atan2(Vz, (Vx^2 + Vy^2)^(1/2)))/pi))/180)*(Vx^2 + Vy^2)^(1/2))/pi))/Iyy;

== matlab function B5_simulation_paparazzi/Model Block Normal Filters/Force and Moment Calculation/Drag Plate Aerodynamics/drag plate My1 ==
  data: w_plate input; h_plate input; l_plate input; theta input; Vx input; Cd output; Cl output; Vx output; Vy output; Vy input; Vz input; Vz output; gamma output; theta output; alpha output; D_plate output; L_plate output; R_plate output; u input; My_dp output
function [Cd,Cl,Vx,Vy,Vz,gamma,theta,alpha,D_plate,L_plate,R_plate,My_dp] = drag_plate_My(w_plate,h_plate,l_plate,theta,Vx,Vy,Vz,u)

% define constants
rho = 1.225;
S_plate = w_plate*h_plate;

% Resultant
Vr = sqrt(Vx^2+Vy^2+Vz^2);
Vh = sqrt(Vx^2+Vy^2);

gamma = -rad2deg(atan2(Vz,Vh));
theta = rad2deg(theta);

alpha = theta-gamma;

% Drag Coefficient
Cd = 0.0033*(90+alpha)+0.7;

% Lift Coefficient
Cl = -0.0228*(90+alpha)+2.01;

% get drag and lift
D_plate= 0.5*rho*Vr^2*S_plate*Cd;
L_plate = 0.5*rho*Vr^2*S_plate*Cl;
R_plate = cos(deg2rad(alpha))*D_plate - sin(deg2rad(alpha))*L_plate;

My_dp = l_plate*R_plate*sign(u);

== matlab function B5_simulation_paparazzi/Model Block Normal Filters/Force and Moment Calculation/Forces due to thrust ==
  data: omega input; R_bg input; G1 input; F_t_e output; F_t_b output
function [F_t_e,F_t_b] = F_t(omega,R_bg,G1)

F_t_b = G1(4,:) * omega;

F_t_vect = [0 0 F_t_b];

F_t_e = R_bg * F_t_vect';

== matlab function B5_simulation_paparazzi/Model Block Normal Filters/Force and Moment Calculation/Moments due to thrust ==
  data: omega input; omega_dot input; M_t output; G1 input; G2 input; sampling_time input; I input
function M_t = M_t(omega, omega_dot, G1, G2, sampling_time, I)

% M_t = I * (G1(1:3,:) * omega + sampling_time * G2 * omega_dot);
M_t = I * (G1(1:3,:) * omega);

== matlab function B5_simulation_paparazzi/Model Block Normal Filters/Plant and State Estimation/Plant Dynamics Continuous/body_to_ground_transorm ==
  data: Phi input; R_bg output; Theta input; Psi input
function R_bg  = R_bg(Phi,Theta,Psi)

% conventional rotation body to ground [312] or ZXY
% R_bg_312 = R_theta * R_phi * R_psi;
R_bg = [cos(Psi)*cos(Theta) cos(Psi)*sin(Phi)*sin(Theta) - cos(Phi)*sin(Psi) sin(Phi)*sin(Psi) + cos(Phi)*cos(Psi)*sin(Theta);
cos(Theta)*sin(Psi) cos(Phi)*cos(Psi) + sin(Phi)*sin(Psi)*sin(Theta) cos(Phi)*sin(Psi)*sin(Theta) - cos(Psi)*sin(Phi);
-sin(Theta) cos(Theta)*sin(Phi) cos(Phi)*cos(Theta)];

== matlab function B5_simulation_paparazzi/Model Block Complementary Filters/Extended INDI/8-shape trajectory/MATLAB Function ==
  data: x output; t input; y output; f input; scale input; psi output; sampling_time input; total_time input; start_time input
function [x,y,psi] = inf_trajectory(t,f,scale,sampling_time,total_time,start_time)

t_norm = t/total_time;

x = 2*scale*sin(2*pi*f*t_norm);
y = scale*sin(2*pi*f*t_norm*2);

x_n = 2*scale*sin(2*pi*f*(t_norm+sampling_time));
y_n = scale*sin(2*pi*f*(t_norm+sampling_time)*2);

dx = x_n - x;
dy = y_n - y;

psi = atan2(dy,dx);

== matlab function B5_simulation_paparazzi/Model Block Complementary Filters/Extended INDI/ERROR CONTROLLER ATTITUDE/MATLAB Function1 ==
  data: pis_e input; psie_w output
function psie_w = wrapper(pis_e)

if pis_e > pi
    psie_w = pis_e - 2*pi;
elseif pis_e <= -pi
    psie_w = pis_e + 2*pi;
else
    psie_w = pis_e;
end

== matlab function B5_simulation_paparazzi/Model Block Normal Filters/Plant and State Estimation/Plant Dynamics Continuous/euler_rates_to_pqr ==
  data: Phi input; R output; Theta input
function R = euler_rates_to_pqr(Phi,Theta)
R = [1 0 -sin(Theta);
0 cos(Phi) cos(Theta)*sin(Phi);
0 -sin(Phi) cos(Phi)*cos(Theta)];

== matlab function B5_simulation_paparazzi/Model Block Normal Filters/Plant and State Estimation/Plant Dynamics Continuous/pqr_to_euler_rates ==
  data: Phi input; T output; Theta input
function T = pqr_to_euler_rates(Phi,Theta)
T = [1 (sin(Phi)*sin(Theta))/cos(Theta) (cos(Phi)*sin(Theta))/cos(Theta);
0 cos(Phi) -sin(Phi);
0 sin(Phi)/cos(Theta) cos(Phi)/cos(Theta)];

== matlab function B5_simulation_paparazzi/Model Block Normal Filters/Plant and State Estimation/Plant Dynamics Continuous/wrapper ==
  data: pis_e input; psie_w output
function psie_w = wrapper(pis_e)

if pis_e > pi
    psie_w = pis_e - 2*pi;
elseif pis_e <= -pi
    psie_w = pis_e + 2*pi;
else
    psie_w = pis_e;
end

== matlab function B5_simulation_paparazzi/Model Block Normal Filters/Plant and State Estimation/body_to_ground_transorm ==
  data: Phi input; R_bg output; Theta input; Psi input
function R_bg  = R_bg(Phi,Theta,Psi)

% conventional rotation body to ground [312] or ZXY
% R_bg_312 = R_theta * R_phi * R_psi;
R_bg = [cos(Psi)*cos(Theta) cos(Psi)*sin(Phi)*sin(Theta) - cos(Phi)*sin(Psi) sin(Phi)*sin(Psi) + cos(Phi)*cos(Psi)*sin(Theta);
cos(Theta)*sin(Psi) cos(Phi)*cos(Psi) + sin(Phi)*sin(Psi)*sin(Theta) cos(Phi)*sin(Psi)*sin(Theta) - cos(Psi)*sin(Phi);
-sin(Theta) cos(Theta)*sin(Phi) cos(Phi)*cos(Theta)];

== matlab function B5_simulation_paparazzi/Model Block Normal Filters/Plant and State Estimation/euler_rates_to_pqr ==
  data: Phi input; R output; Theta input
function R = euler_rates_to_pqr(Phi,Theta)
R = [1 0 -sin(Theta);
0 cos(Phi) cos(Theta)*sin(Phi);
0 -sin(Phi) cos(Phi)*cos(Theta)];

== matlab function B5_simulation_paparazzi/Model Block Normal Filters/Plant and State Estimation/pqr_to_euler_rates ==
  data: Phi input; T output; Theta input
function T = pqr_to_euler_rates(Phi,Theta)
T = [1 (sin(Phi)*sin(Theta))/cos(Theta) (cos(Phi)*sin(Theta))/cos(Theta);
0 cos(Phi) -sin(Phi);
0 sin(Phi)/cos(Theta) cos(Phi)/cos(Theta)];

== matlab function B5_simulation_paparazzi/Model Block Normal Filters/Plant and State Estimation/wrapper ==
  data: pis_e input; psie_w output
function psie_w = wrapper(pis_e)

if pis_e > pi
    psie_w = pis_e - 2*pi;
elseif pis_e <= -pi
    psie_w = pis_e + 2*pi;
else
    psie_w = pis_e;
end

== matlab function B5_simulation_paparazzi/Model Block Normal Filters/Plant and State Estimation/wrapper1 ==
  data: pis_e input; psie_w output
function psie_w = wrapper(pis_e)

if pis_e > pi
    psie_w = pis_e - 2*pi;
elseif pis_e <= -pi
    psie_w = pis_e + 2*pi;
else
    psie_w = pis_e;
end

== matlab function B5_simulation_paparazzi/Model Block Normal Filters/Simple INDI/8-shape trajectory/MATLAB Function ==
  data: x output; t input; y output; f input; scale input; psi output; sampling_time input; total_time input; start_time input
function [x,y,psi] = inf_trajectory(t,f,scale,sampling_time,total_time,start_time)

t_norm = t/total_time;

x = 2*scale*sin(2*pi*f*t_norm);
y = scale*sin(2*pi*f*t_norm*2);

x_n = 2*scale*sin(2*pi*f*(t_norm+sampling_time));
y_n = scale*sin(2*pi*f*(t_norm+sampling_time)*2);

dx = x_n - x;
dy = y_n - y;

psi = atan2(dy,dx);

== matlab function B5_simulation_paparazzi/Model Block Normal Filters/Simple INDI/ERROR CONTROLLER ATTITUDE/MATLAB Function1 ==
  data: pis_e input; psie_w output
function psie_w = wrapper(pis_e)

if pis_e > pi
    psie_w = pis_e - 2*pi;
elseif pis_e <= -pi
    psie_w = pis_e + 2*pi;
else
    psie_w = pis_e;
end

== matlab function B5_simulation_paparazzi/Model Block Normal Filters/Simple INDI/G1+G2 ==
  data: G1 input; B_inner output; G2 input
function B_inner = B_inner(G1,G2)

% add additional row to G2 for equal size
G2_T = [0 0 0 0];
G2 = vertcat(G2,G2_T);

% B_inner = K_act*(G1 + G2);
B_inner = G1;

== matlab function B5_simulation_paparazzi/Model Block Normal Filters/Simple INDI/G2_comp ==
  data: G2 input; domega input; G2_comp output
function G2_comp = G2_comp(G2,domega)

G2_comp = G2(3,:) * domega;

== matlab function B5_simulation_paparazzi/Model Block Complementary Filters/Plant and State Estimation/Angular Velocity Model/Moments due to thrust ==
  data: omega input; omega_dot input; M_t output; G1 input; G2 input; sampling_time input; I input
function M_t = M_t(omega, omega_dot, G1, G2, sampling_time, I)

% M_t = I * (G1(1:3,:) * omega + sampling_time * G2 * omega_dot);
M_t = I * (G1(1:3,:) * omega);

== matlab function B5_simulation_paparazzi/Model Block Normal Filters/Simple INDI/INTERNAL REFERENCE MODEL ATTITUDE/MATLAB Function1 ==
  data: pis_e input; psie_w output
function psie_w = wrapper(pis_e)

if pis_e > pi
    psie_w = pis_e - 2*pi;
elseif pis_e <= -pi
    psie_w = pis_e + 2*pi;
else
    psie_w = pis_e;
end

== matlab function B5_simulation_paparazzi/Model Block Normal Filters/Simple INDI/MATLAB Function1 ==
  data: T input; B_outer output; Phi input; Theta input; Psi input; m input
function B_outer = control_allocation_simple_outer(T,Phi,Theta,Psi,m)

B_outer = zeros(3,3);

% matrix obtained in ZXY rotation
% output order u = [phi theta thrust]
B_outer(1,1) = (T*cos(Phi)*cos(Psi)*cos(Theta))/m;
B_outer(2,1) = (T*cos(Phi)*cos(Theta)*sin(Psi))/m;
B_outer(3,1) = -(T*cos(Phi)*sin(Theta))/m;

B_outer(1,2) = (T*(cos(Phi)*sin(Psi) - cos(Psi)*sin(Phi)*sin(Theta)))/m;
B_outer(2,2) = -(T*(cos(Phi)*cos(Psi) + sin(Phi)*sin(Psi)*sin(Theta)))/m;
B_outer(3,2) = -(T*cos(Theta)*sin(Phi))/m;

B_outer(1,3) = (sin(Phi)*sin(Psi) + cos(Phi)*cos(Psi)*sin(Theta))/m;
B_outer(2,3) = -(cos(Psi)*sin(Phi) - cos(Phi)*sin(Psi)*sin(Theta))/m;
B_outer(3,3) = (cos(Phi)*cos(Theta))/m;

end

== matlab function B5_simulation_paparazzi/Model Block Complementary Filters/Extended INDI/G1+G2 ==
  data: G1 input; B_inner output; G2 input; K_act input
function B_inner = B_inner(G1,G2,K_act)

% add additional row to G2 for equal size
G2_T = [0 0 0 0];
G2 = vertcat(G2,G2_T);

B_inner = K_act*(G1 + G2);
% B_inner = K_act*(G1);

== matlab function B5_simulation_paparazzi/Model Block Complementary Filters/Extended INDI/G2_comp ==
  data: G2 input; K_act input; domega input; G2_comp output
function G2_comp = G2_comp(G2,K_act,domega)

G2_comp = K_act * G2(3,:) * domega;

== matlab function B5_simulation_paparazzi/Model Block Complementary Filters/Extended INDI/INTERNAL REFERENCE MODEL ATTITUDE/MATLAB Function1 ==
  data: pis_e input; psie_w output
function psie_w = wrapper(pis_e)

if pis_e > pi
    psie_w = pis_e - 2*pi;
elseif pis_e <= -pi
    psie_w = pis_e + 2*pi;
else
    psie_w = pis_e;
end

== matlab function B5_simulation_paparazzi/Model Block Complementary Filters/Extended INDI/MATLAB Function1 ==
  data: T input; B_outer output; Phi input; Theta input; Psi input; m input
function B_outer = control_allocation_simple_outer(T,Phi,Theta,Psi,m)

B_outer = zeros(3,3);

% matrix obtained in ZXY rotation
% output order u = [phi theta thrust]
B_outer(1,1) = (T*cos(Phi)*cos(Psi)*cos(Theta))/m;
B_outer(2,1) = (T*cos(Phi)*cos(Theta)*sin(Psi))/m;
B_outer(3,1) = -(T*cos(Phi)*sin(Theta))/m;

B_outer(1,2) = (T*(cos(Phi)*sin(Psi) - cos(Psi)*sin(Phi)*sin(Theta)))/m;
B_outer(2,2) = -(T*(cos(Phi)*cos(Psi) + sin(Phi)*sin(Psi)*sin(Theta)))/m;
B_outer(3,2) = -(T*cos(Theta)*sin(Phi))/m;

B_outer(1,3) = (sin(Phi)*sin(Psi) + cos(Phi)*cos(Psi)*sin(Theta))/m;
B_outer(2,3) = -(cos(Psi)*sin(Phi) - cos(Phi)*sin(Psi)*sin(Theta))/m;
B_outer(3,3) = (cos(Phi)*cos(Theta))/m;

end

== matlab function B5_simulation_paparazzi/Model Block Complementary Filters/Force and Moment Calculation/Forces due to thrust ==
  data: omega input; R_bg input; G1 input; F_t_e output; F_t_b output
function [F_t_e,F_t_b] = F_t(omega,R_bg,G1)

F_t_b = G1(4,:) * omega;

F_t_vect = [0 0 F_t_b];

F_t_e = R_bg * F_t_vect';

== matlab function B5_simulation_paparazzi/Model Block Complementary Filters/Force and Moment Calculation/Moments due to thrust ==
  data: omega input; omega_dot input; M_t output; G1 input; G2 input; sampling_time input; I input
function M_t = M_t(omega, omega_dot, G1, G2, sampling_time, I)

M_t = I * (G1(1:3,:) * omega + sampling_time * G2 * omega_dot);
% M_t = I * (G1(1:3,:) * omega);

== matlab function B5_simulation_paparazzi/Model Block Complementary Filters/Plant and State Estimation/Plant Dynamics Continuous/body_to_ground_transorm ==
  data: Phi input; R_bg output; Theta input; Psi input
function R_bg  = R_bg(Phi,Theta,Psi)

% conventional rotation body to ground [312] or ZXY
% R_bg_312 = R_theta * R_phi * R_psi;
R_bg = [cos(Psi)*cos(Theta) cos(Psi)*sin(Phi)*sin(Theta) - cos(Phi)*sin(Psi) sin(Phi)*sin(Psi) + cos(Phi)*cos(Psi)*sin(Theta);
cos(Theta)*sin(Psi) cos(Phi)*cos(Psi) + sin(Phi)*sin(Psi)*sin(Theta) cos(Phi)*sin(Psi)*sin(Theta) - cos(Psi)*sin(Phi);
-sin(Theta) cos(Theta)*sin(Phi) cos(Phi)*cos(Theta)];

== matlab function B5_simulation_paparazzi/Model Block Complementary Filters/Plant and State Estimation/Plant Dynamics Continuous/euler_rates_to_pqr ==
  data: Phi input; R output; Theta input
function R = euler_rates_to_pqr(Phi,Theta)
R = [1 0 -sin(Theta);
0 cos(Phi) cos(Theta)*sin(Phi);
0 -sin(Phi) cos(Phi)*cos(Theta)];

== matlab function B5_simulation_paparazzi/Model Block Complementary Filters/Plant and State Estimation/Plant Dynamics Continuous/pqr_to_euler_rates ==
  data: Phi input; T output; Theta input
function T = pqr_to_euler_rates(Phi,Theta)
T = [1 (sin(Phi)*sin(Theta))/cos(Theta) (cos(Phi)*sin(Theta))/cos(Theta);
0 cos(Phi) -sin(Phi);
0 sin(Phi)/cos(Theta) cos(Phi)/cos(Theta)];

== matlab function B5_simulation_paparazzi/Model Block Complementary Filters/Plant and State Estimation/Plant Dynamics Continuous/wrapper ==
  data: pis_e input; psie_w output
function psie_w = wrapper(pis_e)

if pis_e > pi
    psie_w = pis_e - 2*pi;
elseif pis_e <= -pi
    psie_w = pis_e + 2*pi;
else
    psie_w = pis_e;
end

== matlab function B5_simulation_paparazzi/Model Block Complementary Filters/Plant and State Estimation/body_to_ground_transorm ==
  data: Phi input; R_bg output; Theta input; Psi input
function R_bg  = R_bg(Phi,Theta,Psi)

% conventional rotation body to ground [312] or ZXY
% R_bg_312 = R_theta * R_phi * R_psi;
R_bg = [cos(Psi)*cos(Theta) cos(Psi)*sin(Phi)*sin(Theta) - cos(Phi)*sin(Psi) sin(Phi)*sin(Psi) + cos(Phi)*cos(Psi)*sin(Theta);
cos(Theta)*sin(Psi) cos(Phi)*cos(Psi) + sin(Phi)*sin(Psi)*sin(Theta) cos(Phi)*sin(Psi)*sin(Theta) - cos(Psi)*sin(Phi);
-sin(Theta) cos(Theta)*sin(Phi) cos(Phi)*cos(Theta)];

== matlab function B5_simulation_paparazzi/Model Block Complementary Filters/Plant and State Estimation/euler_rates_to_pqr ==
  data: Phi input; R output; Theta input
function R = euler_rates_to_pqr(Phi,Theta)
R = [1 0 -sin(Theta);
0 cos(Phi) cos(Theta)*sin(Phi);
0 -sin(Phi) cos(Phi)*cos(Theta)];

== matlab function B5_simulation_paparazzi/Model Block Complementary Filters/Plant and State Estimation/Angular Velocity Model/Drag Plate Aerodynamics/drag plate My1 ==
  data: w_plate input; h_plate input; l_plate input; theta input; Vx input; Cd output; Cl output; Vx output; Vy output; Vy input; Vz input; Vz output; gamma output; theta output; alpha output; D_plate output; L_plate output; R_plate output; u input; My_dp output
function [Cd,Cl,Vx,Vy,Vz,gamma,theta,alpha,D_plate,L_plate,R_plate,My_dp] = drag_plate_My(w_plate,h_plate,l_plate,theta,Vx,Vy,Vz,u)

% define constants
rho = 1.225;
S_plate = w_plate*h_plate;

% Resultant
Vr = sqrt(Vx^2+Vy^2+Vz^2);
Vh = sqrt(Vx^2+Vy^2);

gamma = -rad2deg(atan2(Vz,Vh));
theta = rad2deg(theta);

alpha = theta-gamma;

% Drag Coefficient
Cd = 0.0033*(90+alpha)+0.7;

% Lift Coefficient
Cl = -0.0228*(90+alpha)+2.01;

% get drag and lift
D_plate= 0.5*rho*Vr^2*S_plate*Cd;
L_plate = 0.5*rho*Vr^2*S_plate*Cl;
R_plate = cos(deg2rad(alpha))*D_plate - sin(deg2rad(alpha))*L_plate;

My_dp = l_plate*R_plate*sign(u);

== matlab function B5_simulation_paparazzi/Model Block Complementary Filters/Plant and State Estimation/pqr_to_euler_rates ==
  data: Phi input; T output; Theta input
function T = pqr_to_euler_rates(Phi,Theta)
T = [1 (sin(Phi)*sin(Theta))/cos(Theta) (cos(Phi)*sin(Theta))/cos(Theta);
0 cos(Phi) -sin(Phi);
0 sin(Phi)/cos(Theta) cos(Phi)/cos(Theta)];

== matlab function B5_simulation_paparazzi/Model Block Complementary Filters/Plant and State Estimation/wrapper ==
  data: pis_e input; psie_w output
function psie_w = wrapper(pis_e)

if pis_e > pi
    psie_w = pis_e - 2*pi;
elseif pis_e <= -pi
    psie_w = pis_e + 2*pi;
else
    psie_w = pis_e;
end

== matlab function B5_simulation_paparazzi/Model Block Complementary Filters/Plant and State Estimation/wrapper1 ==
  data: pis_e input; psie_w output
function psie_w = wrapper(pis_e)

if pis_e > pi
    psie_w = pis_e - 2*pi;
elseif pis_e <= -pi
    psie_w = pis_e + 2*pi;
else
    psie_w = pis_e;
end

== matlab function B5_simulation_paparazzi/Model Block Complementary Filters/Plant and State Estimation/Subsystem1/Forces due to thrust ==
  data: omega_1 input; omega_2 input; F_t_e output; omega_3 input; omega_4 input; R_bg input; K_t input; F_t_b output
function [F_t_e,F_t_b] = F_t(omega_1, omega_2, omega_3, omega_4, R_bg, K_t)

f_1 = [0 0 -K_t * omega_1^2];
f_2 = [0 0 -K_t * omega_2^2]; 
f_3 = [0 0 -K_t * omega_3^2]; 
f_4 = [0 0 -K_t * omega_4^2];

F_t_e = R_bg * (f_1' + f_2' + f_3' + f_4');
F_t_b = (f_1(:,3) + f_2(:,3) + f_3(:,3) + f_4(:,3));
